simulink model "final_heart_sym2_level5_hdl"  (R2021a)
settings: Solver=FixedStepDiscrete  StartTime=0.0  StopTime=10.0  RelTol=1e-3
undefined symbols (not defined in the file or in its folder): lambda2
(part 2 of 3)

== system final_heart_sym2_level5_hdl/DWT_Sym2_Level5/1st_Level_Decomp4/HiD_Even ==
  In_HiD_e : Inport  OutDataTypeStr=fixdt(0,16,24)  SampleTime=1/44100
  Add : Sum  AccumDataTypeStr=fixdt(1,16,15)  OutDataTypeStr=fixdt(1,16,15)
  Delay : Delay  DelayLength=1  SampleTime=1/44100
  Delay3 : Delay  DelayLength=1  SampleTime=1/44100
  HiD_0 : Constant  Value=-0.482962913  OutDataTypeStr=fixdt(1,16,16)  SampleTime=1/44100
  HiD_2 : Constant  Value=-0.224143868  OutDataTypeStr=fixdt(1,16,17)  SampleTime=1/44100
  Multiply : Product  OutDataTypeStr=fixdt(1,16,15)
  Multiply1 : Product  OutDataTypeStr=fixdt(1,16,15)
  Rate Transition : RateTransition
  Out_HiD_e : Outport  OutDataTypeStr=fixdt(1,16,15)  SampleTime=1/44100  VectorParamsAs1DForOutWhenUnconnected=off
  wires:
  Delay/1 -> Rate Transition/1
  Delay3/1 -> Add/2
  Multiply1/1 -> Delay3/1
  Multiply/1 -> Add/1
  HiD_0/1 -> Multiply/1
  HiD_2/1 -> Multiply1/1
  Add/1 -> Out_HiD_e/1
  In_HiD_e/1 -> Multiply/2, Delay/1
  Rate Transition/1 -> Multiply1/2

== system final_heart_sym2_level5_hdl/DWT_Sym2_Level5/1st_Level_Decomp4/HiD_Odd ==
  In_HiD_o : Inport  OutDataTypeStr=fixdt(0,16,24)  SampleTime=1/44100
  Add : Sum  AccumDataTypeStr=fixdt(1,16,23)  OutDataTypeStr=fixdt(1,16,24)
  Delay : Delay  DelayLength=1  SampleTime=1/44100
  Delay3 : Delay  DelayLength=1  SampleTime=1/44100
  HiD_1 : Constant  Value=0.836516304  OutDataTypeStr=fixdt(0,16,16)  SampleTime=1/44100
  HiD_3 : Constant  Value=-0.129409523  OutDataTypeStr=fixdt(1,16,17)  SampleTime=1/44100
  Multiply : Product  OutDataTypeStr=fixdt(0,16,24)
  Multiply1 : Product  OutDataTypeStr=fixdt(1,16,15)
  Rate Transition : RateTransition
  Out_HiD_o : Outport  OutDataTypeStr=fixdt(1,16,24)  SampleTime=1/44100  VectorParamsAs1DForOutWhenUnconnected=off
  wires:
  Delay/1 -> Rate Transition/1
  Delay3/1 -> Add/2
  Multiply1/1 -> Delay3/1
  Multiply/1 -> Add/1
  HiD_1/1 -> Multiply/1
  HiD_3/1 -> Multiply1/1
  Add/1 -> Out_HiD_o/1
  In_HiD_o/1 -> Delay/1, Multiply/2
  Rate Transition/1 -> Multiply1/2

== system final_heart_sym2_level5_hdl/DWT_Sym2_Level5/1st_Level_Decomp4/LoD_Even ==
  In_LoD_e : Inport  OutDataTypeStr=fixdt(0,16,24)  SampleTime=1/44100
  Add : Sum  AccumDataTypeStr=fixdt(1,16,23)  OutDataTypeStr=fixdt(1,16,24)
  Delay : Delay  DelayLength=1  SampleTime=1/44100
  Delay3 : Delay  DelayLength=1  SampleTime=1/44100
  LoD_0 : Constant  Value=-0.129409523  OutDataTypeStr=fixdt(1,16,17)  SampleTime=1/44100
  LoD_2 : Constant  Value=0.836516304  OutDataTypeStr=fixdt(0,16,16)  SampleTime=1/44100
  Multiply : Product  OutDataTypeStr=fixdt(1,16,15)
  Multiply1 : Product  OutDataTypeStr=fixdt(0,16,24)
  Rate Transition : RateTransition
  Out_LoD_e : Outport  OutDataTypeStr=fixdt(1,16,24)  SampleTime=1/44100  VectorParamsAs1DForOutWhenUnconnected=off
  wires:
  Delay/1 -> Rate Transition/1
  Delay3/1 -> Add/2
  Multiply1/1 -> Delay3/1
  Multiply/1 -> Add/1
  LoD_0/1 -> Multiply/1
  LoD_2/1 -> Multiply1/1
  Add/1 -> Out_LoD_e/1
  In_LoD_e/1 -> Delay/1, Multiply/2
  Rate Transition/1 -> Multiply1/2

== system final_heart_sym2_level5_hdl/DWT_Sym2_Level5/1st_Level_Decomp4/LoD_Odd ==
  In_LoD_o : Inport  OutDataTypeStr=fixdt(0,16,24)  SampleTime=1/44100
  Add : Sum  AccumDataTypeStr=fixdt(0,16,25)  OutDataTypeStr=fixdt(0,16,25)
  Delay : Delay  DelayLength=1  SampleTime=1/44100
  Delay3 : Delay  DelayLength=1  SampleTime=1/44100
  LoD_1 : Constant  Value=0.224143868  OutDataTypeStr=fixdt(0,16,18)  SampleTime=1/44100
  LoD_3 : Constant  Value=0.482962913  OutDataTypeStr=fixdt(0,16,17)  SampleTime=1/44100
  Multiply : Product  OutDataTypeStr=fixdt(0,16,26)
  Multiply1 : Product  OutDataTypeStr=fixdt(0,16,25)
  Rate Transition : RateTransition
  Out_LoD_o : Outport  OutDataTypeStr=fixdt(0,16,25)  SampleTime=1/44100  VectorParamsAs1DForOutWhenUnconnected=off
  wires:
  Delay/1 -> Rate Transition/1
  Delay3/1 -> Add/2
  Multiply1/1 -> Delay3/1
  Multiply/1 -> Add/1
  LoD_1/1 -> Multiply/1
  LoD_3/1 -> Multiply1/1
  Add/1 -> Out_LoD_o/1
  In_LoD_o/1 -> Delay/1, Multiply/2
  Rate Transition/1 -> Multiply1/2

== system final_heart_sym2_level5_hdl/DWT_Sym2_Level5/1st_Level_Recon/HiR_Even ==
  In_HiR_e : Inport  OutDataTypeStr=fixdt(1,16,27)  SampleTime=1/44100
  Add : Sum  AccumDataTypeStr=fixdt(1,16,28)  OutDataTypeStr=fixdt(1,16,28)
  Constant12 : Constant  Value=-0.129409523  OutDataTypeStr=fixdt(1,16,17)  SampleTime=1/44100
  Constant14 : Constant  Value=0.836516304  OutDataTypeStr=fixdt(0,16,16)  SampleTime=1/44100
  Delay : Delay  DelayLength=1  SampleTime=1/44100
  Delay3 : Delay  DelayLength=1  SampleTime=1/44100
  Multiply : Product  OutDataTypeStr=fixdt(1,16,30)
  Multiply1 : Product  OutDataTypeStr=fixdt(1,16,28)
  Rate Transition : RateTransition
  Out_HiR_e : Outport  OutDataTypeStr=fixdt(1,16,28)  SampleTime=1/44100  VectorParamsAs1DForOutWhenUnconnected=off
  wires:
  In_HiR_e/1 -> Multiply/2, Delay/1
  Delay3/1 -> Add/2
  Multiply/1 -> Add/1
  Constant12/1 -> Multiply/1
  Constant14/1 -> Multiply1/1
  Delay/1 -> Rate Transition/1
  Multiply1/1 -> Delay3/1
  Add/1 -> Out_HiR_e/1
  Rate Transition/1 -> Multiply1/2

== system final_heart_sym2_level5_hdl/DWT_Sym2_Level5/1st_Level_Recon/HiR_Odd ==
  In_HiR_o : Inport  OutDataTypeStr=fixdt(1,16,27)  SampleTime=1/44100
  Add : Sum  AccumDataTypeStr=fixdt(1,16,29)  OutDataTypeStr=fixdt(1,16,29)
  Constant13 : Constant  Value=-0.224143868  OutDataTypeStr=fixdt(1,16,17)  SampleTime=1/44100
  Constant15 : Constant  Value=-0.482962913  OutDataTypeStr=fixdt(1,16,16)  SampleTime=1/44100
  Delay : Delay  DelayLength=1  SampleTime=1/44100
  Delay3 : Delay  DelayLength=1  SampleTime=1/44100
  Multiply : Product  OutDataTypeStr=fixdt(1,16,30)
  Multiply1 : Product  OutDataTypeStr=fixdt(1,16,29)
  Rate Transition : RateTransition
  Out_HiR_o : Outport  OutDataTypeStr=fixdt(1,16,29)  SampleTime=1/44100  VectorParamsAs1DForOutWhenUnconnected=off
  wires:
  In_HiR_o/1 -> Multiply/2, Delay/1
  Delay3/1 -> Add/2
  Multiply1/1 -> Delay3/1
  Multiply/1 -> Add/1
  Constant13/1 -> Multiply/1
  Constant15/1 -> Multiply1/1
  Add/1 -> Out_HiR_o/1
  Delay/1 -> Rate Transition/1
  Rate Transition/1 -> Multiply1/2

== system final_heart_sym2_level5_hdl/DWT_Sym2_Level5/1st_Level_Recon/LoR_Even ==
  In_LoR_e : Inport  OutDataTypeStr=fixdt(0,16,24)  SampleTime=1/44100
  Add : Sum  AccumDataTypeStr=fixdt(0,16,25)  OutDataTypeStr=fixdt(0,16,25)
  Constant10 : Constant  Value=0.224143868  OutDataTypeStr=fixdt(0,16,18)  SampleTime=1/44100
  Constant8 : Constant  Value=0.482962913  OutDataTypeStr=fixdt(0,16,17)  SampleTime=1/44100
  Delay : Delay  DelayLength=1  SampleTime=1/44100
  Delay3 : Delay  DelayLength=1  SampleTime=1/44100
  Multiply : Product  OutDataTypeStr=fixdt(0,16,25)
  Multiply1 : Product  OutDataTypeStr=fixdt(0,16,27)
  Rate Transition : RateTransition
  Out_LoR_e : Outport  OutDataTypeStr=fixdt(0,16,25)  SampleTime=1/44100  VectorParamsAs1DForOutWhenUnconnected=off
  wires:
  In_LoR_e/1 -> Multiply/2, Delay/1
  Delay3/1 -> Add/2
  Multiply1/1 -> Delay3/1
  Multiply/1 -> Add/1
  Constant8/1 -> Multiply/1
  Constant10/1 -> Multiply1/1
  Add/1 -> Out_LoR_e/1
  Delay/1 -> Rate Transition/1
  Rate Transition/1 -> Multiply1/2

== system final_heart_sym2_level5_hdl/DWT_Sym2_Level5/1st_Level_Recon/LoR_Odd ==
  In_LoR_o : Inport  OutDataTypeStr=fixdt(0,16,24)  SampleTime=1/44100
  Add : Sum  AccumDataTypeStr=fixdt(1,16,24)  OutDataTypeStr=fixdt(1,16,24)
  Constant11 : Constant  Value=-0.129409523  OutDataTypeStr=fixdt(1,16,17)  SampleTime=1/44100
  Constant9 : Constant  Value=0.836516304  OutDataTypeStr=fixdt(0,16,16)  SampleTime=1/44100
  Delay : Delay  DelayLength=1  SampleTime=1/44100
  Delay3 : Delay  DelayLength=1  SampleTime=1/44100
  Multiply : Product  OutDataTypeStr=fixdt(0,16,25)
  Multiply1 : Product  OutDataTypeStr=fixdt(1,16,15)
  Rate Transition : RateTransition
  Out_HiR_o : Outport  OutDataTypeStr=fixdt(1,16,24)  SampleTime=1/44100  VectorParamsAs1DForOutWhenUnconnected=off
  wires:
  In_LoR_o/1 -> Multiply/2, Delay/1
  Delay3/1 -> Add/2
  Multiply1/1 -> Delay3/1
  Multiply/1 -> Add/1
  Constant9/1 -> Multiply/1
  Constant11/1 -> Multiply1/1
  Add/1 -> Out_HiR_o/1
  Delay/1 -> Rate Transition/1
  Rate Transition/1 -> Multiply1/2

== system final_heart_sym2_level5_hdl/DWT_Sym2_Level5/1st_Level_Recon1/HiR_Even ==
  In_HiR_e : Inport  OutDataTypeStr=fixdt(1,16,27)  SampleTime=1/44100
  Add : Sum  AccumDataTypeStr=fixdt(1,16,28)  OutDataTypeStr=fixdt(1,16,28)
  Constant12 : Constant  Value=-0.129409523  OutDataTypeStr=fixdt(1,16,17)  SampleTime=1/44100
  Constant14 : Constant  Value=0.836516304  OutDataTypeStr=fixdt(0,16,16)  SampleTime=1/44100
  Delay : Delay  DelayLength=1  SampleTime=1/44100
  Delay3 : Delay  DelayLength=1  SampleTime=1/44100
  Multiply : Product  OutDataTypeStr=fixdt(1,16,30)
  Multiply1 : Product  OutDataTypeStr=fixdt(1,16,28)
  Rate Transition : RateTransition
  Out_HiR_e : Outport  OutDataTypeStr=fixdt(1,16,28)  SampleTime=1/44100  VectorParamsAs1DForOutWhenUnconnected=off
  wires:
  In_HiR_e/1 -> Multiply/2, Delay/1
  Delay3/1 -> Add/2
  Multiply/1 -> Add/1
  Constant12/1 -> Multiply/1
  Constant14/1 -> Multiply1/1
  Delay/1 -> Rate Transition/1
  Multiply1/1 -> Delay3/1
  Add/1 -> Out_HiR_e/1
  Rate Transition/1 -> Multiply1/2

== system final_heart_sym2_level5_hdl/DWT_Sym2_Level5/1st_Level_Recon1/HiR_Odd ==
  In_HiR_o : Inport  OutDataTypeStr=fixdt(1,16,27)  SampleTime=1/44100
  Add : Sum  AccumDataTypeStr=fixdt(1,16,29)  OutDataTypeStr=fixdt(1,16,29)
  Constant13 : Constant  Value=-0.224143868  OutDataTypeStr=fixdt(1,16,17)  SampleTime=1/44100
  Constant15 : Constant  Value=-0.482962913  OutDataTypeStr=fixdt(1,16,16)  SampleTime=1/44100
  Delay : Delay  DelayLength=1  SampleTime=1/44100
  Delay3 : Delay  DelayLength=1  SampleTime=1/44100
  Multiply : Product  OutDataTypeStr=fixdt(1,16,30)
  Multiply1 : Product  OutDataTypeStr=fixdt(1,16,29)
  Rate Transition : RateTransition
  Out_HiR_o : Outport  OutDataTypeStr=fixdt(1,16,29)  SampleTime=1/44100  VectorParamsAs1DForOutWhenUnconnected=off
  wires:
  In_HiR_o/1 -> Multiply/2, Delay/1
  Delay3/1 -> Add/2
  Multiply1/1 -> Delay3/1
  Multiply/1 -> Add/1
  Constant13/1 -> Multiply/1
  Constant15/1 -> Multiply1/1
  Add/1 -> Out_HiR_o/1
  Delay/1 -> Rate Transition/1
  Rate Transition/1 -> Multiply1/2

== system final_heart_sym2_level5_hdl/DWT_Sym2_Level5/1st_Level_Recon1/LoR_Even ==
  In_LoR_e : Inport  OutDataTypeStr=fixdt(1,16,23)  SampleTime=1/44100
  Add : Sum  AccumDataTypeStr=fixdt(1,16,24)  OutDataTypeStr=fixdt(1,16,24)
  Constant10 : Constant  Value=0.224143868  OutDataTypeStr=fixdt(0,16,18)  SampleTime=1/44100
  Constant8 : Constant  Value=0.482962913  OutDataTypeStr=fixdt(0,16,17)  SampleTime=1/44100
  Delay : Delay  DelayLength=1  SampleTime=1/44100
  Delay3 : Delay  DelayLength=1  SampleTime=1/44100
  Multiply : Product  OutDataTypeStr=fixdt(1,16,24)
  Multiply1 : Product  OutDataTypeStr=fixdt(1,16,25)
  Rate Transition : RateTransition
  Out_LoR_e : Outport  OutDataTypeStr=fixdt(1,16,24)  SampleTime=1/44100  VectorParamsAs1DForOutWhenUnconnected=off
  wires:
  In_LoR_e/1 -> Multiply/2, Delay/1
  Delay3/1 -> Add/2
  Multiply1/1 -> Delay3/1
  Multiply/1 -> Add/1
  Constant8/1 -> Multiply/1
  Constant10/1 -> Multiply1/1
  Add/1 -> Out_LoR_e/1
  Delay/1 -> Rate Transition/1
  Rate Transition/1 -> Multiply1/2

== system final_heart_sym2_level5_hdl/DWT_Sym2_Level5/1st_Level_Recon1/LoR_Odd ==
  In_LoR_o : Inport  OutDataTypeStr=fixdt(1,16,23)  SampleTime=1/44100
  Add : Sum  AccumDataTypeStr=fixdt(1,16,23)  OutDataTypeStr=fixdt(1,16,24)
  Constant11 : Constant  Value=-0.129409523  OutDataTypeStr=fixdt(1,16,17)  SampleTime=1/44100
  Constant9 : Constant  Value=0.836516304  OutDataTypeStr=fixdt(0,16,16)  SampleTime=1/44100
  Delay : Delay  DelayLength=1  SampleTime=1/44100
  Delay3 : Delay  DelayLength=1  SampleTime=1/44100
  Multiply : Product  OutDataTypeStr=fixdt(1,16,23)
  Multiply1 : Product  OutDataTypeStr=fixdt(1,16,26)
  Rate Transition : RateTransition
  Out_HiR_o : Outport  OutDataTypeStr=fixdt(1,16,24)  SampleTime=1/44100  VectorParamsAs1DForOutWhenUnconnected=off
  wires:
  In_LoR_o/1 -> Multiply/2, Delay/1
  Delay3/1 -> Add/2
  Multiply1/1 -> Delay3/1
  Multiply/1 -> Add/1
  Constant9/1 -> Multiply/1
  Constant11/1 -> Multiply1/1
  Add/1 -> Out_HiR_o/1
  Delay/1 -> Rate Transition/1
  Rate Transition/1 -> Multiply1/2

== system final_heart_sym2_level5_hdl/DWT_Sym2_Level5/1st_Level_Recon2/HiR_Even ==
  In_HiR_e : Inport  OutDataTypeStr=fixdt(1,16,27)  SampleTime=1/44100
  Add : Sum  AccumDataTypeStr=fixdt(1,16,28)  OutDataTypeStr=fixdt(1,16,28)
  Constant12 : Constant  Value=-0.129409523  OutDataTypeStr=fixdt(1,16,17)  SampleTime=1/44100
  Constant14 : Constant  Value=0.836516304  OutDataTypeStr=fixdt(0,16,16)  SampleTime=1/44100
  Delay : Delay  DelayLength=1  SampleTime=1/44100
  Delay3 : Delay  DelayLength=1  SampleTime=1/44100
  Multiply : Product  OutDataTypeStr=fixdt(1,16,30)
  Multiply1 : Product  OutDataTypeStr=fixdt(1,16,28)
  Rate Transition : RateTransition
  Out_HiR_e : Outport  OutDataTypeStr=fixdt(1,16,28)  SampleTime=1/44100  VectorParamsAs1DForOutWhenUnconnected=off
  wires:
  In_HiR_e/1 -> Multiply/2, Delay/1
  Delay3/1 -> Add/2
  Multiply/1 -> Add/1
  Constant12/1 -> Multiply/1
  Constant14/1 -> Multiply1/1
  Delay/1 -> Rate Transition/1
  Multiply1/1 -> Delay3/1
  Add/1 -> Out_HiR_e/1
  Rate Transition/1 -> Multiply1/2

== system final_heart_sym2_level5_hdl/DWT_Sym2_Level5/1st_Level_Recon2/HiR_Odd ==
  In_HiR_o : Inport  OutDataTypeStr=fixdt(1,16,27)  SampleTime=1/44100
  Add : Sum  AccumDataTypeStr=fixdt(1,16,29)  OutDataTypeStr=fixdt(1,16,29)
  Constant13 : Constant  Value=-0.224143868  OutDataTypeStr=fixdt(1,16,17)  SampleTime=1/44100
  Constant15 : Constant  Value=-0.482962913  OutDataTypeStr=fixdt(1,16,16)  SampleTime=1/44100
  Delay : Delay  DelayLength=1  SampleTime=1/44100
  Delay3 : Delay  DelayLength=1  SampleTime=1/44100
  Multiply : Product  OutDataTypeStr=fixdt(1,16,30)
  Multiply1 : Product  OutDataTypeStr=fixdt(1,16,29)
  Rate Transition : RateTransition
  Out_HiR_o : Outport  OutDataTypeStr=fixdt(1,16,29)  SampleTime=1/44100  VectorParamsAs1DForOutWhenUnconnected=off
  wires:
  In_HiR_o/1 -> Multiply/2, Delay/1
  Delay3/1 -> Add/2
  Multiply1/1 -> Delay3/1
  Multiply/1 -> Add/1
  Constant13/1 -> Multiply/1
  Constant15/1 -> Multiply1/1
  Add/1 -> Out_HiR_o/1
  Delay/1 -> Rate Transition/1
  Rate Transition/1 -> Multiply1/2

== system final_heart_sym2_level5_hdl/DWT_Sym2_Level5/1st_Level_Recon2/LoR_Even ==
  In_LoR_e : Inport  OutDataTypeStr=fixdt(1,16,23)  SampleTime=1/44100
  Add : Sum  AccumDataTypeStr=fixdt(1,16,23)  OutDataTypeStr=fixdt(1,16,23)
  Constant10 : Constant  Value=0.224143868  OutDataTypeStr=fixdt(0,16,18)  SampleTime=1/44100
  Constant8 : Constant  Value=0.482962913  OutDataTypeStr=fixdt(0,16,17)  SampleTime=1/44100
  Delay : Delay  DelayLength=1  SampleTime=1/44100
  Delay3 : Delay  DelayLength=1  SampleTime=1/44100
  Multiply : Product  OutDataTypeStr=fixdt(1,16,24)
  Multiply1 : Product  OutDataTypeStr=fixdt(1,16,25)
  Rate Transition : RateTransition
  Out_LoR_e : Outport  OutDataTypeStr=fixdt(1,16,23)  SampleTime=1/44100  VectorParamsAs1DForOutWhenUnconnected=off
  wires:
  In_LoR_e/1 -> Multiply/2, Delay/1
  Delay3/1 -> Add/2
  Multiply1/1 -> Delay3/1
  Multiply/1 -> Add/1
  Constant8/1 -> Multiply/1
  Constant10/1 -> Multiply1/1
  Add/1 -> Out_LoR_e/1
  Delay/1 -> Rate Transition/1
  Rate Transition/1 -> Multiply1/2

== system final_heart_sym2_level5_hdl/DWT_Sym2_Level5/1st_Level_Recon2/LoR_Odd ==
  In_LoR_o : Inport  OutDataTypeStr=fixdt(1,16,23)  SampleTime=1/44100
  Add : Sum  AccumDataTypeStr=fixdt(1,16,23)  OutDataTypeStr=fixdt(1,16,23)
  Constant11 : Constant  Value=-0.129409523  OutDataTypeStr=fixdt(1,16,17)  SampleTime=1/44100
  Constant9 : Constant  Value=0.836516304  OutDataTypeStr=fixdt(0,16,16)  SampleTime=1/44100
  Delay : Delay  DelayLength=1  SampleTime=1/44100
  Delay3 : Delay  DelayLength=1  SampleTime=1/44100
  Multiply : Product  OutDataTypeStr=fixdt(1,16,23)
  Multiply1 : Product  OutDataTypeStr=fixdt(1,16,26)
  Rate Transition : RateTransition
  Out_HiR_o : Outport  OutDataTypeStr=fixdt(1,16,23)  SampleTime=1/44100  VectorParamsAs1DForOutWhenUnconnected=off
  wires:
  In_LoR_o/1 -> Multiply/2, Delay/1
  Delay3/1 -> Add/2
  Multiply1/1 -> Delay3/1
  Multiply/1 -> Add/1
  Constant9/1 -> Multiply/1
  Constant11/1 -> Multiply1/1
  Add/1 -> Out_HiR_o/1
  Delay/1 -> Rate Transition/1
  Rate Transition/1 -> Multiply1/2

== system final_heart_sym2_level5_hdl/DWT_Sym2_Level5/1st_Level_Recon3/HiR_Even ==
  In_HiR_e : Inport  OutDataTypeStr=fixdt(1,16,27)  SampleTime=1/44100
  Add : Sum  AccumDataTypeStr=fixdt(1,16,28)  OutDataTypeStr=fixdt(1,16,28)
  Constant12 : Constant  Value=-0.129409523  OutDataTypeStr=fixdt(1,16,17)  SampleTime=1/44100
  Constant14 : Constant  Value=0.836516304  OutDataTypeStr=fixdt(0,16,16)  SampleTime=1/44100
  Delay : Delay  DelayLength=1  SampleTime=1/44100
  Delay3 : Delay  DelayLength=1  SampleTime=1/44100
  Multiply : Product  OutDataTypeStr=fixdt(1,16,30)
  Multiply1 : Product  OutDataTypeStr=fixdt(1,16,28)
  Rate Transition : RateTransition
  Out_HiR_e : Outport  OutDataTypeStr=fixdt(1,16,28)  SampleTime=1/44100  VectorParamsAs1DForOutWhenUnconnected=off
  wires:
  In_HiR_e/1 -> Multiply/2, Delay/1
  Delay3/1 -> Add/2
  Multiply/1 -> Add/1
  Constant12/1 -> Multiply/1
  Constant14/1 -> Multiply1/1
  Delay/1 -> Rate Transition/1
  Multiply1/1 -> Delay3/1
  Add/1 -> Out_HiR_e/1
  Rate Transition/1 -> Multiply1/2

== system final_heart_sym2_level5_hdl/DWT_Sym2_Level5/1st_Level_Recon3/HiR_Odd ==
  In_HiR_o : Inport  OutDataTypeStr=fixdt(1,16,27)  SampleTime=1/44100
  Add : Sum  AccumDataTypeStr=fixdt(1,16,29)  OutDataTypeStr=fixdt(1,16,29)
  Constant13 : Constant  Value=-0.224143868  OutDataTypeStr=fixdt(1,16,17)  SampleTime=1/44100
  Constant15 : Constant  Value=-0.482962913  OutDataTypeStr=fixdt(1,16,16)  SampleTime=1/44100
  Delay : Delay  DelayLength=1  SampleTime=1/44100
  Delay3 : Delay  DelayLength=1  SampleTime=1/44100
  Multiply : Product  OutDataTypeStr=fixdt(1,16,30)
  Multiply1 : Product  OutDataTypeStr=fixdt(1,16,29)
  Rate Transition : RateTransition
  Out_HiR_o : Outport  OutDataTypeStr=fixdt(1,16,29)  SampleTime=1/44100  VectorParamsAs1DForOutWhenUnconnected=off
  wires:
  In_HiR_o/1 -> Multiply/2, Delay/1
  Delay3/1 -> Add/2
  Multiply1/1 -> Delay3/1
  Multiply/1 -> Add/1
  Constant13/1 -> Multiply/1
  Constant15/1 -> Multiply1/1
  Add/1 -> Out_HiR_o/1
  Delay/1 -> Rate Transition/1
  Rate Transition/1 -> Multiply1/2

== system final_heart_sym2_level5_hdl/DWT_Sym2_Level5/1st_Level_Recon3/LoR_Even ==
  In_LoR_e : Inport  OutDataTypeStr=fixdt(1,16,23)  SampleTime=1/44100
  Add : Sum  AccumDataTypeStr=fixdt(1,16,23)  OutDataTypeStr=fixdt(1,16,23)
  Constant10 : Constant  Value=0.224143868  OutDataTypeStr=fixdt(0,16,18)  SampleTime=1/44100
  Constant8 : Constant  Value=0.482962913  OutDataTypeStr=fixdt(0,16,17)  SampleTime=1/44100
  Delay : Delay  DelayLength=1  SampleTime=1/44100
  Delay3 : Delay  DelayLength=1  SampleTime=1/44100
  Multiply : Product  OutDataTypeStr=fixdt(1,16,24)
  Multiply1 : Product  OutDataTypeStr=fixdt(1,16,25)
  Rate Transition : RateTransition
  Out_LoR_e : Outport  OutDataTypeStr=fixdt(1,16,23)  SampleTime=1/44100  VectorParamsAs1DForOutWhenUnconnected=off
  wires:
  In_LoR_e/1 -> Multiply/2, Delay/1
  Delay3/1 -> Add/2
  Multiply1/1 -> Delay3/1
  Multiply/1 -> Add/1
  Constant8/1 -> Multiply/1
  Constant10/1 -> Multiply1/1
  Add/1 -> Out_LoR_e/1
  Delay/1 -> Rate Transition/1
  Rate Transition/1 -> Multiply1/2

== system final_heart_sym2_level5_hdl/DWT_Sym2_Level5/1st_Level_Recon3/LoR_Odd ==
  In_LoR_o : Inport  OutDataTypeStr=fixdt(1,16,23)  SampleTime=1/44100
  Add : Sum  AccumDataTypeStr=fixdt(1,16,23)  OutDataTypeStr=fixdt(1,16,23)
  Constant11 : Constant  Value=-0.129409523  OutDataTypeStr=fixdt(1,16,17)  SampleTime=1/44100
  Constant9 : Constant  Value=0.836516304  OutDataTypeStr=fixdt(0,16,16)  SampleTime=1/44100
  Delay : Delay  DelayLength=1  SampleTime=1/44100
  Delay3 : Delay  DelayLength=1  SampleTime=1/44100
  Multiply : Product  OutDataTypeStr=fixdt(1,16,23)
  Multiply1 : Product  OutDataTypeStr=fixdt(1,16,26)
  Rate Transition : RateTransition
  Out_HiR_o : Outport  OutDataTypeStr=fixdt(1,16,23)  SampleTime=1/44100  VectorParamsAs1DForOutWhenUnconnected=off
  wires:
  In_LoR_o/1 -> Multiply/2, Delay/1
  Delay3/1 -> Add/2
  Multiply1/1 -> Delay3/1
  Multiply/1 -> Add/1
  Constant9/1 -> Multiply/1
  Constant11/1 -> Multiply1/1
  Add/1 -> Out_HiR_o/1
  Delay/1 -> Rate Transition/1
  Rate Transition/1 -> Multiply1/2

== system final_heart_sym2_level5_hdl/DWT_Sym2_Level5/1st_Level_Recon4/HiR_Even ==
  In_HiR_e : Inport  OutDataTypeStr=fixdt(1,16,28)  SampleTime=1/44100
  Add : Sum  AccumDataTypeStr=fixdt(1,16,28)  OutDataTypeStr=fixdt(1,16,28)
  Constant12 : Constant  Value=-0.129409523  OutDataTypeStr=fixdt(1,16,17)  SampleTime=1/44100
  Constant14 : Constant  Value=0.836516304  OutDataTypeStr=fixdt(0,16,16)  SampleTime=1/44100
  Delay : Delay  DelayLength=1  SampleTime=1/44100
  Delay3 : Delay  DelayLength=1  SampleTime=1/44100
  Multiply : Product  OutDataTypeStr=fixdt(1,16,30)
  Multiply1 : Product  OutDataTypeStr=fixdt(1,16,28)
  Rate Transition : RateTransition
  Out_HiR_e : Outport  OutDataTypeStr=fixdt(1,16,28)  SampleTime=1/44100  VectorParamsAs1DForOutWhenUnconnected=off
  wires:
  In_HiR_e/1 -> Multiply/2, Delay/1
  Delay3/1 -> Add/2
  Multiply/1 -> Add/1
  Constant12/1 -> Multiply/1
  Constant14/1 -> Multiply1/1
  Delay/1 -> Rate Transition/1
  Multiply1/1 -> Delay3/1
  Add/1 -> Out_HiR_e/1
  Rate Transition/1 -> Multiply1/2

== system final_heart_sym2_level5_hdl/DWT_Sym2_Level5/1st_Level_Recon4/HiR_Odd ==
  In_HiR_o : Inport  OutDataTypeStr=fixdt(1,16,28)  SampleTime=1/44100
  Add : Sum  AccumDataTypeStr=fixdt(1,16,28)  OutDataTypeStr=fixdt(1,16,28)
  Constant13 : Constant  Value=-0.224143868  OutDataTypeStr=fixdt(1,16,17)  SampleTime=1/44100
  Constant15 : Constant  Value=-0.482962913  OutDataTypeStr=fixdt(1,16,16)  SampleTime=1/44100
  Delay : Delay  DelayLength=1  SampleTime=1/44100
  Delay3 : Delay  DelayLength=1  SampleTime=1/44100
  Multiply : Product  OutDataTypeStr=fixdt(1,16,30)
  Multiply1 : Product  OutDataTypeStr=fixdt(1,16,29)
  Rate Transition : RateTransition
  Out_HiR_o : Outport  OutDataTypeStr=fixdt(1,16,28)  SampleTime=1/44100  VectorParamsAs1DForOutWhenUnconnected=off
  wires:
  In_HiR_o/1 -> Multiply/2, Delay/1
  Delay3/1 -> Add/2
  Multiply1/1 -> Delay3/1
  Multiply/1 -> Add/1
  Constant13/1 -> Multiply/1
  Constant15/1 -> Multiply1/1
  Add/1 -> Out_HiR_o/1
  Delay/1 -> Rate Transition/1
  Rate Transition/1 -> Multiply1/2

== system final_heart_sym2_level5_hdl/DWT_Sym2_Level5/1st_Level_Recon4/LoR_Even ==
  In_LoR_e : Inport  OutDataTypeStr=fixdt(1,16,22)  SampleTime=1/44100
  Add : Sum  AccumDataTypeStr=fixdt(1,16,23)  OutDataTypeStr=fixdt(1,16,23)
  Constant10 : Constant  Value=0.224143868  OutDataTypeStr=fixdt(0,16,18)  SampleTime=1/44100
  Constant8 : Constant  Value=0.482962913  OutDataTypeStr=fixdt(0,16,17)  SampleTime=1/44100
  Delay : Delay  DelayLength=1  SampleTime=1/44100
  Delay3 : Delay  DelayLength=1  SampleTime=1/44100
  Multiply : Product  OutDataTypeStr=fixdt(1,16,23)
  Multiply1 : Product  OutDataTypeStr=fixdt(1,16,25)
  Rate Transition : RateTransition
  Out_LoR_e : Outport  OutDataTypeStr=fixdt(1,16,23)  SampleTime=1/44100  VectorParamsAs1DForOutWhenUnconnected=off
  wires:
  In_LoR_e/1 -> Multiply/2, Delay/1
  Delay3/1 -> Add/2
  Multiply1/1 -> Delay3/1
  Multiply/1 -> Add/1
  Constant8/1 -> Multiply/1
  Constant10/1 -> Multiply1/1
  Add/1 -> Out_LoR_e/1
  Delay/1 -> Rate Transition/1
  Rate Transition/1 -> Multiply1/2

== system final_heart_sym2_level5_hdl/DWT_Sym2_Level5/1st_Level_Recon4/LoR_Odd ==
  In_LoR_o : Inport  OutDataTypeStr=fixdt(1,16,22)  SampleTime=1/44100
  Add : Sum  AccumDataTypeStr=fixdt(1,16,23)  OutDataTypeStr=fixdt(1,16,23)
  Constant11 : Constant  Value=-0.129409523  OutDataTypeStr=fixdt(1,16,17)  SampleTime=1/44100
  Constant9 : Constant  Value=0.836516304  OutDataTypeStr=fixdt(0,16,16)  SampleTime=1/44100
  Delay : Delay  DelayLength=1  SampleTime=1/44100
  Delay3 : Delay  DelayLength=1  SampleTime=1/44100
  Multiply : Product  OutDataTypeStr=fixdt(1,16,23)
  Multiply1 : Product  OutDataTypeStr=fixdt(1,16,25)
  Rate Transition : RateTransition
  Out_HiR_o : Outport  OutDataTypeStr=fixdt(1,16,23)  SampleTime=1/44100  VectorParamsAs1DForOutWhenUnconnected=off
  wires:
  In_LoR_o/1 -> Multiply/2, Delay/1
  Delay3/1 -> Add/2
  Multiply1/1 -> Delay3/1
  Multiply/1 -> Add/1
  Constant9/1 -> Multiply/1
  Constant11/1 -> Multiply1/1
  Add/1 -> Out_HiR_o/1
  Delay/1 -> Rate Transition/1
  Rate Transition/1 -> Multiply1/2

== system final_heart_sym2_level5_hdl/DWT_Sym2_Level5/Threshold_Estimator/Absolute_Value1 ==
  Signal_w4 : Inport  OutDataTypeStr=fixdt(1,16,26)  SampleTime=1/44100
  Absolute_Switch : Switch  Threshold=1  OutDataTypeStr=fixdt(0,16,27)
  Constant295 : Constant  Value=0  OutDataTypeStr=fixdt(1,16,4)  SampleTime=1/44100
  Gain2 : Gain  Gain=-1  ParamDataTypeStr=fixdt(1,16,15)  OutDataTypeStr=fixdt(0,16,28)
  Relational Operator2 : RelationalOperator  Operator=<  OutDataTypeStr=boolean  RndMeth=Simplest
  Out_Abs : Outport  OutDataTypeStr=fixdt(0,16,27)  SampleTime=1/44100  VectorParamsAs1DForOutWhenUnconnected=off
  wires:
  Absolute_Switch/1 -> Out_Abs/1
  Relational Operator2/1 -> Absolute_Switch/2
  Gain2/1 -> Absolute_Switch/1
  Signal_w4/1 -> Absolute_Switch/3, Relational Operator2/1, Gain2/1
  Constant295/1 -> Relational Operator2/2

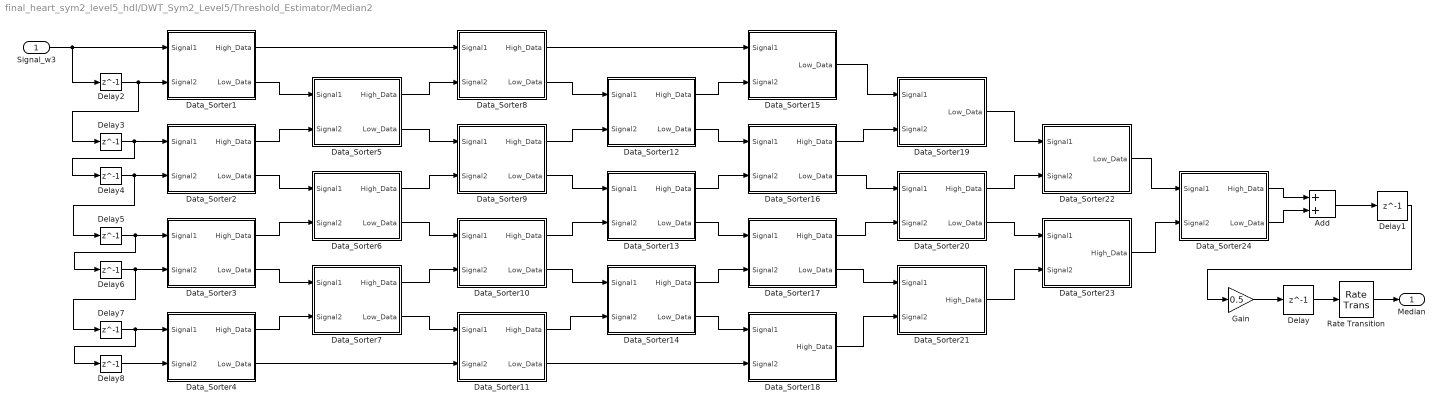
== system final_heart_sym2_level5_hdl/DWT_Sym2_Level5/Threshold_Estimator/Median2 ==
  Signal_w3 : Inport  OutDataTypeStr=fixdt(0,16,27)  SampleTime=1/44100
  Add : Sum  AccumDataTypeStr=fixdt(0,16,26)  OutDataTypeStr=fixdt(0,16,26)
  Data_Sorter1 : Subsystem
  Data_Sorter10 : Subsystem
  Data_Sorter11 : Subsystem
  Data_Sorter12 : Subsystem
  Data_Sorter13 : Subsystem
  Data_Sorter14 : Subsystem
  Data_Sorter15 : Subsystem
  Data_Sorter16 : Subsystem
  Data_Sorter17 : Subsystem
  Data_Sorter18 : Subsystem
  Data_Sorter19 : Subsystem
  Data_Sorter2 : Subsystem
  Data_Sorter20 : Subsystem
  Data_Sorter21 : Subsystem
  Data_Sorter22 : Subsystem
  Data_Sorter23 : Subsystem
  Data_Sorter24 : Subsystem
  Data_Sorter3 : Subsystem
  Data_Sorter4 : Subsystem
  Data_Sorter5 : Subsystem
  Data_Sorter6 : Subsystem
  Data_Sorter7 : Subsystem
  Data_Sorter8 : Subsystem
  Data_Sorter9 : Subsystem
  Delay{,1..8} (9 alike) : Delay  DelayLength=1  SampleTime=1/44100
  Gain : Gain  Gain=0.5  ParamDataTypeStr=fixdt(0,16,16)  OutDataTypeStr=fixdt(0,16,27)
  Rate Transition : RateTransition
  Median : Outport  OutDataTypeStr=fixdt(0,16,27)  SampleTime=1/44100  VectorParamsAs1DForOutWhenUnconnected=off
  wires:
  Data_Sorter4/1(High_Data) -> Data_Sorter7/2(Signal2)
  Delay3/1 -> Data_Sorter2/1(Signal1), Delay4/1
  Signal_w3/1 -> Data_Sorter1/1(Signal1), Delay2/1
  Data_Sorter10/1(High_Data) -> Data_Sorter13/2(Signal2)
  Data_Sorter23/1(High_Data) -> Data_Sorter24/2(Signal2)
  Data_Sorter12/2(Low_Data) -> Data_Sorter16/1(Signal1)
  Delay2/1 -> Delay3/1, Data_Sorter1/2(Signal2)
  Data_Sorter5/1(High_Data) -> Data_Sorter8/2(Signal2)
  Delay/1 -> Rate Transition/1
  Data_Sorter15/1(Low_Data) -> Data_Sorter19/1(Signal1)
  Add/1 -> Delay1/1
  Data_Sorter7/2(Low_Data) -> Data_Sorter11/1(Signal1)
  Data_Sorter24/1(High_Data) -> Add/1
  Data_Sorter1/2(Low_Data) -> Data_Sorter5/1(Signal1)
  Data_Sorter3/1(High_Data) -> Data_Sorter6/2(Signal2)
  Data_Sorter22/1(Low_Data) -> Data_Sorter24/1(Signal1)
  Data_Sorter2/1(High_Data) -> Data_Sorter5/2(Signal2)
  Data_Sorter10/2(Low_Data) -> Data_Sorter14/1(Signal1)
  Delay1/1 -> Gain/1
  Data_Sorter17/2(Low_Data) -> Data_Sorter21/1(Signal1)
  Data_Sorter21/1(High_Data) -> Data_Sorter23/2(Signal2)
  Data_Sorter7/1(High_Data) -> Data_Sorter10/2(Signal2)
  Delay4/1 -> Data_Sorter2/2(Signal2), Delay5/1
  Data_Sorter16/1(High_Data) -> Data_Sorter19/2(Signal2)
  Data_Sorter20/1(High_Data) -> Data_Sorter22/2(Signal2)
  Data_Sorter16/2(Low_Data) -> Data_Sorter20/1(Signal1)
  Data_Sorter3/2(Low_Data) -> Data_Sorter7/1(Signal1)
  Data_Sorter2/2(Low_Data) -> Data_Sorter6/1(Signal1)
  Data_Sorter6/2(Low_Data) -> Data_Sorter10/1(Signal1)
  Data_Sorter19/1(Low_Data) -> Data_Sorter22/1(Signal1)
  Data_Sorter12/1(High_Data) -> Data_Sorter15/2(Signal2)
  Data_Sorter5/2(Low_Data) -> Data_Sorter9/1(Signal1)
  Data_Sorter24/2(Low_Data) -> Add/2
  Data_Sorter17/1(High_Data) -> Data_Sorter20/2(Signal2)
  Data_Sorter13/1(High_Data) -> Data_Sorter16/2(Signal2)
  Data_Sorter11/1(High_Data) -> Data_Sorter14/2(Signal2)
  Delay8/1 -> Data_Sorter4/2(Signal2)
  Data_Sorter8/2(Low_Data) -> Data_Sorter12/1(Signal1)
  Delay6/1 -> Data_Sorter3/2(Signal2), Delay7/1
  Data_Sorter9/2(Low_Data) -> Data_Sorter13/1(Signal1)
  Data_Sorter4/2(Low_Data) -> Data_Sorter11/2(Signal2)
  Data_Sorter9/1(High_Data) -> Data_Sorter12/2(Signal2)
  Data_Sorter14/2(Low_Data) -> Data_Sorter18/1(Signal1)
  Delay5/1 -> Data_Sorter3/1(Signal1), Delay6/1
  Delay7/1 -> Data_Sorter4/1(Signal1), Delay8/1
  Data_Sorter1/1(High_Data) -> Data_Sorter8/1(Signal1)
  Data_Sorter8/1(High_Data) -> Data_Sorter15/1(Signal1)
  Data_Sorter14/1(High_Data) -> Data_Sorter17/2(Signal2)
  Data_Sorter6/1(High_Data) -> Data_Sorter9/2(Signal2)
  Data_Sorter20/2(Low_Data) -> Data_Sorter23/1(Signal1)
  Data_Sorter11/2(Low_Data) -> Data_Sorter18/2(Signal2)
  Data_Sorter13/2(Low_Data) -> Data_Sorter17/1(Signal1)
  Gain/1 -> Delay/1
  Data_Sorter18/1(High_Data) -> Data_Sorter21/2(Signal2)
  Rate Transition/1 -> Median/1

== system final_heart_sym2_level5_hdl/DWT_Sym2_Level5/Threshold_Estimator/Median2/Data_Sorter1 ==
  Signal1 : Inport  OutDataTypeStr=fixdt(0,16,27)  SampleTime=1/44100
  Signal2 : Inport  Port=2  OutDataTypeStr=fixdt(0,16,27)  SampleTime=1/44100
  Data_Sorter_Switch : Switch  OutDataTypeStr=fixdt(0,16,27)
  Data_Sorter_Switch1 : Switch  Threshold=1  OutDataTypeStr=fixdt(0,16,27)
  Delay1 : Delay  DelayLength=1  SampleTime=1/44100
  Delay2 : Delay  DelayLength=1  SampleTime=1/44100
  Relational Operator2 : RelationalOperator  Operator=<  OutDataTypeStr=boolean  RndMeth=Simplest
  High_Data : Outport  OutDataTypeStr=fixdt(0,16,27)  SampleTime=1/44100  VectorParamsAs1DForOutWhenUnconnected=off
  Low_Data : Outport  Port=2  OutDataTypeStr=fixdt(0,16,27)  SampleTime=1/44100  VectorParamsAs1DForOutWhenUnconnected=off
  wires:
  Signal1/1 -> Data_Sorter_Switch/3, Data_Sorter_Switch/1, Relational Operator2/1
  Relational Operator2/1 -> Data_Sorter_Switch1/2, Data_Sorter_Switch/2
  Signal2/1 -> Data_Sorter_Switch1/1, Data_Sorter_Switch1/3, Relational Operator2/2
  Data_Sorter_Switch1/1 -> Delay2/1
  Delay2/1 -> Low_Data/1
  Data_Sorter_Switch/1 -> Delay1/1
  Delay1/1 -> High_Data/1

== system final_heart_sym2_level5_hdl/DWT_Sym2_Level5/Threshold_Estimator/Median2/Data_Sorter10 ==
  Signal1 : Inport  OutDataTypeStr=fixdt(0,16,27)  SampleTime=1/44100
  Signal2 : Inport  Port=2  OutDataTypeStr=fixdt(0,16,27)  SampleTime=1/44100
  Data_Sorter_Switch : Switch  OutDataTypeStr=fixdt(0,16,27)
  Data_Sorter_Switch1 : Switch  Threshold=1  OutDataTypeStr=fixdt(0,16,27)
  Delay1 : Delay  DelayLength=1  SampleTime=1/44100
  Delay2 : Delay  DelayLength=1  SampleTime=1/44100
  Relational Operator2 : RelationalOperator  Operator=<  OutDataTypeStr=boolean  RndMeth=Simplest
  High_Data : Outport  OutDataTypeStr=fixdt(0,16,27)  SampleTime=1/44100  VectorParamsAs1DForOutWhenUnconnected=off
  Low_Data : Outport  Port=2  OutDataTypeStr=fixdt(0,16,27)  SampleTime=1/44100  VectorParamsAs1DForOutWhenUnconnected=off
  wires:
  Signal1/1 -> Data_Sorter_Switch/3, Data_Sorter_Switch/1, Relational Operator2/1
  Relational Operator2/1 -> Data_Sorter_Switch1/2, Data_Sorter_Switch/2
  Signal2/1 -> Data_Sorter_Switch1/1, Data_Sorter_Switch1/3, Relational Operator2/2
  Data_Sorter_Switch1/1 -> Delay2/1
  Delay2/1 -> Low_Data/1
  Data_Sorter_Switch/1 -> Delay1/1
  Delay1/1 -> High_Data/1

== system final_heart_sym2_level5_hdl/DWT_Sym2_Level5/Threshold_Estimator/Median2/Data_Sorter11 ==
  Signal1 : Inport  OutDataTypeStr=fixdt(0,16,27)  SampleTime=1/44100
  Signal2 : Inport  Port=2  OutDataTypeStr=fixdt(0,16,27)  SampleTime=1/44100
  Data_Sorter_Switch : Switch  OutDataTypeStr=fixdt(0,16,27)
  Data_Sorter_Switch1 : Switch  Threshold=1  OutDataTypeStr=fixdt(0,16,27)
  Delay1 : Delay  DelayLength=1  SampleTime=1/44100
  Delay2 : Delay  DelayLength=1  SampleTime=1/44100
  Relational Operator2 : RelationalOperator  Operator=<  OutDataTypeStr=boolean  RndMeth=Simplest
  High_Data : Outport  OutDataTypeStr=fixdt(0,16,27)  SampleTime=1/44100  VectorParamsAs1DForOutWhenUnconnected=off
  Low_Data : Outport  Port=2  OutDataTypeStr=fixdt(0,16,27)  SampleTime=1/44100  VectorParamsAs1DForOutWhenUnconnected=off
  wires:
  Signal1/1 -> Data_Sorter_Switch/3, Data_Sorter_Switch/1, Relational Operator2/1
  Relational Operator2/1 -> Data_Sorter_Switch1/2, Data_Sorter_Switch/2
  Signal2/1 -> Data_Sorter_Switch1/1, Data_Sorter_Switch1/3, Relational Operator2/2
  Data_Sorter_Switch1/1 -> Delay2/1
  Delay2/1 -> Low_Data/1
  Data_Sorter_Switch/1 -> Delay1/1
  Delay1/1 -> High_Data/1

== system final_heart_sym2_level5_hdl/DWT_Sym2_Level5/Threshold_Estimator/Median2/Data_Sorter12 ==
  Signal1 : Inport  OutDataTypeStr=fixdt(0,16,27)  SampleTime=1/44100
  Signal2 : Inport  Port=2  OutDataTypeStr=fixdt(0,16,27)  SampleTime=1/44100
  Data_Sorter_Switch : Switch  OutDataTypeStr=fixdt(0,16,27)
  Data_Sorter_Switch1 : Switch  Threshold=1  OutDataTypeStr=fixdt(0,16,27)
  Delay1 : Delay  DelayLength=1  SampleTime=1/44100
  Delay2 : Delay  DelayLength=1  SampleTime=1/44100
  Relational Operator2 : RelationalOperator  Operator=<  OutDataTypeStr=boolean  RndMeth=Simplest
  High_Data : Outport  OutDataTypeStr=fixdt(0,16,27)  SampleTime=1/44100  VectorParamsAs1DForOutWhenUnconnected=off
  Low_Data : Outport  Port=2  OutDataTypeStr=fixdt(0,16,27)  SampleTime=1/44100  VectorParamsAs1DForOutWhenUnconnected=off
  wires:
  Signal1/1 -> Data_Sorter_Switch/3, Data_Sorter_Switch/1, Relational Operator2/1
  Relational Operator2/1 -> Data_Sorter_Switch1/2, Data_Sorter_Switch/2
  Signal2/1 -> Data_Sorter_Switch1/1, Data_Sorter_Switch1/3, Relational Operator2/2
  Data_Sorter_Switch1/1 -> Delay2/1
  Delay2/1 -> Low_Data/1
  Data_Sorter_Switch/1 -> Delay1/1
  Delay1/1 -> High_Data/1

== system final_heart_sym2_level5_hdl/DWT_Sym2_Level5/Threshold_Estimator/Median2/Data_Sorter13 ==
  Signal1 : Inport  OutDataTypeStr=fixdt(0,16,27)  SampleTime=1/44100
  Signal2 : Inport  Port=2  OutDataTypeStr=fixdt(0,16,27)  SampleTime=1/44100
  Data_Sorter_Switch : Switch  OutDataTypeStr=fixdt(0,16,27)
  Data_Sorter_Switch1 : Switch  Threshold=1  OutDataTypeStr=fixdt(0,16,27)
  Delay1 : Delay  DelayLength=1  SampleTime=1/44100
  Delay2 : Delay  DelayLength=1  SampleTime=1/44100
  Relational Operator2 : RelationalOperator  Operator=<  OutDataTypeStr=boolean  RndMeth=Simplest
  High_Data : Outport  OutDataTypeStr=fixdt(0,16,27)  SampleTime=1/44100  VectorParamsAs1DForOutWhenUnconnected=off
  Low_Data : Outport  Port=2  OutDataTypeStr=fixdt(0,16,27)  SampleTime=1/44100  VectorParamsAs1DForOutWhenUnconnected=off
  wires:
  Signal1/1 -> Data_Sorter_Switch/3, Data_Sorter_Switch/1, Relational Operator2/1
  Relational Operator2/1 -> Data_Sorter_Switch1/2, Data_Sorter_Switch/2
  Signal2/1 -> Data_Sorter_Switch1/1, Data_Sorter_Switch1/3, Relational Operator2/2
  Data_Sorter_Switch1/1 -> Delay2/1
  Delay2/1 -> Low_Data/1
  Data_Sorter_Switch/1 -> Delay1/1
  Delay1/1 -> High_Data/1

== system final_heart_sym2_level5_hdl/DWT_Sym2_Level5/Threshold_Estimator/Median2/Data_Sorter14 ==
  Signal1 : Inport  OutDataTypeStr=fixdt(0,16,27)  SampleTime=1/44100
  Signal2 : Inport  Port=2  OutDataTypeStr=fixdt(0,16,27)  SampleTime=1/44100
  Data_Sorter_Switch : Switch  OutDataTypeStr=fixdt(0,16,27)
  Data_Sorter_Switch1 : Switch  Threshold=1  OutDataTypeStr=fixdt(0,16,27)
  Delay1 : Delay  DelayLength=1  SampleTime=1/44100
  Delay2 : Delay  DelayLength=1  SampleTime=1/44100
  Relational Operator2 : RelationalOperator  Operator=<  OutDataTypeStr=boolean  RndMeth=Simplest
  High_Data : Outport  OutDataTypeStr=fixdt(0,16,27)  SampleTime=1/44100  VectorParamsAs1DForOutWhenUnconnected=off
  Low_Data : Outport  Port=2  OutDataTypeStr=fixdt(0,16,27)  SampleTime=1/44100  VectorParamsAs1DForOutWhenUnconnected=off
  wires:
  Signal1/1 -> Data_Sorter_Switch/3, Data_Sorter_Switch/1, Relational Operator2/1
  Relational Operator2/1 -> Data_Sorter_Switch1/2, Data_Sorter_Switch/2
  Signal2/1 -> Data_Sorter_Switch1/1, Data_Sorter_Switch1/3, Relational Operator2/2
  Data_Sorter_Switch1/1 -> Delay2/1
  Delay2/1 -> Low_Data/1
  Data_Sorter_Switch/1 -> Delay1/1
  Delay1/1 -> High_Data/1

== system final_heart_sym2_level5_hdl/DWT_Sym2_Level5/Threshold_Estimator/Median2/Data_Sorter15 ==
  Signal1 : Inport  OutDataTypeStr=fixdt(0,16,27)  SampleTime=1/44100
  Signal2 : Inport  Port=2  OutDataTypeStr=fixdt(0,16,27)  SampleTime=1/44100
  Data_Sorter_Switch1 : Switch  Threshold=1  OutDataTypeStr=fixdt(0,16,27)
  Delay2 : Delay  DelayLength=1  SampleTime=1/44100
  Relational Operator2 : RelationalOperator  Operator=<  OutDataTypeStr=boolean  RndMeth=Simplest
  Low_Data : Outport  OutDataTypeStr=fixdt(0,16,27)  SampleTime=1/44100  VectorParamsAs1DForOutWhenUnconnected=off
  wires:
  Signal1/1 -> Relational Operator2/1
  Relational Operator2/1 -> Data_Sorter_Switch1/2
  Signal2/1 -> Data_Sorter_Switch1/1, Data_Sorter_Switch1/3, Relational Operator2/2
  Data_Sorter_Switch1/1 -> Delay2/1
  Delay2/1 -> Low_Data/1

== system final_heart_sym2_level5_hdl/DWT_Sym2_Level5/Threshold_Estimator/Median2/Data_Sorter16 ==
  Signal1 : Inport  OutDataTypeStr=fixdt(0,16,27)  SampleTime=1/44100
  Signal2 : Inport  Port=2  OutDataTypeStr=fixdt(0,16,27)  SampleTime=1/44100
  Data_Sorter_Switch : Switch  OutDataTypeStr=fixdt(0,16,27)
  Data_Sorter_Switch1 : Switch  Threshold=1  OutDataTypeStr=fixdt(0,16,27)
  Delay1 : Delay  DelayLength=1  SampleTime=1/44100
  Delay2 : Delay  DelayLength=1  SampleTime=1/44100
  Relational Operator2 : RelationalOperator  Operator=<  OutDataTypeStr=boolean  RndMeth=Simplest
  High_Data : Outport  OutDataTypeStr=fixdt(0,16,27)  SampleTime=1/44100  VectorParamsAs1DForOutWhenUnconnected=off
  Low_Data : Outport  Port=2  OutDataTypeStr=fixdt(0,16,27)  SampleTime=1/44100  VectorParamsAs1DForOutWhenUnconnected=off
  wires:
  Signal1/1 -> Data_Sorter_Switch/3, Data_Sorter_Switch/1, Relational Operator2/1
  Relational Operator2/1 -> Data_Sorter_Switch1/2, Data_Sorter_Switch/2
  Signal2/1 -> Data_Sorter_Switch1/1, Data_Sorter_Switch1/3, Relational Operator2/2
  Data_Sorter_Switch1/1 -> Delay2/1
  Delay2/1 -> Low_Data/1
  Data_Sorter_Switch/1 -> Delay1/1
  Delay1/1 -> High_Data/1

== system final_heart_sym2_level5_hdl/DWT_Sym2_Level5/Threshold_Estimator/Median2/Data_Sorter17 ==
  Signal1 : Inport  OutDataTypeStr=fixdt(0,16,27)  SampleTime=1/44100
  Signal2 : Inport  Port=2  OutDataTypeStr=fixdt(0,16,27)  SampleTime=1/44100
  Data_Sorter_Switch : Switch  OutDataTypeStr=fixdt(0,16,27)
  Data_Sorter_Switch1 : Switch  Threshold=1  OutDataTypeStr=fixdt(0,16,27)
  Delay1 : Delay  DelayLength=1  SampleTime=1/44100
  Delay2 : Delay  DelayLength=1  SampleTime=1/44100
  Relational Operator2 : RelationalOperator  Operator=<  OutDataTypeStr=boolean  RndMeth=Simplest
  High_Data : Outport  OutDataTypeStr=fixdt(0,16,27)  SampleTime=1/44100  VectorParamsAs1DForOutWhenUnconnected=off
  Low_Data : Outport  Port=2  OutDataTypeStr=fixdt(0,16,27)  SampleTime=1/44100  VectorParamsAs1DForOutWhenUnconnected=off
  wires:
  Signal1/1 -> Data_Sorter_Switch/3, Data_Sorter_Switch/1, Relational Operator2/1
  Relational Operator2/1 -> Data_Sorter_Switch1/2, Data_Sorter_Switch/2
  Signal2/1 -> Data_Sorter_Switch1/1, Data_Sorter_Switch1/3, Relational Operator2/2
  Data_Sorter_Switch1/1 -> Delay2/1
  Delay2/1 -> Low_Data/1
  Data_Sorter_Switch/1 -> Delay1/1
  Delay1/1 -> High_Data/1

== system final_heart_sym2_level5_hdl/DWT_Sym2_Level5/Threshold_Estimator/Median2/Data_Sorter18 ==
  Signal1 : Inport  OutDataTypeStr=fixdt(0,16,27)  SampleTime=1/44100
  Signal2 : Inport  Port=2  OutDataTypeStr=fixdt(0,16,27)  SampleTime=1/44100
  Data_Sorter_Switch : Switch  OutDataTypeStr=fixdt(0,16,27)
  Delay1 : Delay  DelayLength=1  SampleTime=1/44100
  Relational Operator2 : RelationalOperator  Operator=<  OutDataTypeStr=boolean  RndMeth=Simplest
  High_Data : Outport  OutDataTypeStr=fixdt(0,16,27)  SampleTime=1/44100  VectorParamsAs1DForOutWhenUnconnected=off
  wires:
  Signal1/1 -> Data_Sorter_Switch/3, Data_Sorter_Switch/1, Relational Operator2/1
  Relational Operator2/1 -> Data_Sorter_Switch/2
  Signal2/1 -> Relational Operator2/2
  Data_Sorter_Switch/1 -> Delay1/1
  Delay1/1 -> High_Data/1

== system final_heart_sym2_level5_hdl/DWT_Sym2_Level5/Threshold_Estimator/Median2/Data_Sorter19 ==
  Signal1 : Inport  OutDataTypeStr=fixdt(0,16,27)  SampleTime=1/44100
  Signal2 : Inport  Port=2  OutDataTypeStr=fixdt(0,16,27)  SampleTime=1/44100
  Data_Sorter_Switch1 : Switch  Threshold=1  OutDataTypeStr=fixdt(0,16,27)
  Delay2 : Delay  DelayLength=1  SampleTime=1/44100
  Relational Operator2 : RelationalOperator  Operator=<  OutDataTypeStr=boolean  RndMeth=Simplest
  Low_Data : Outport  OutDataTypeStr=fixdt(0,16,27)  SampleTime=1/44100  VectorParamsAs1DForOutWhenUnconnected=off
  wires:
  Signal1/1 -> Relational Operator2/1
  Relational Operator2/1 -> Data_Sorter_Switch1/2
  Signal2/1 -> Data_Sorter_Switch1/1, Data_Sorter_Switch1/3, Relational Operator2/2
  Data_Sorter_Switch1/1 -> Delay2/1
  Delay2/1 -> Low_Data/1

== system final_heart_sym2_level5_hdl/DWT_Sym2_Level5/Threshold_Estimator/Median2/Data_Sorter2 ==
  Signal1 : Inport  OutDataTypeStr=fixdt(0,16,27)  SampleTime=1/44100
  Signal2 : Inport  Port=2  OutDataTypeStr=fixdt(0,16,27)  SampleTime=1/44100
  Data_Sorter_Switch : Switch  OutDataTypeStr=fixdt(0,16,27)
  Data_Sorter_Switch1 : Switch  Threshold=1  OutDataTypeStr=fixdt(0,16,27)
  Delay1 : Delay  DelayLength=1  SampleTime=1/44100
  Delay2 : Delay  DelayLength=1  SampleTime=1/44100
  Relational Operator2 : RelationalOperator  Operator=<  OutDataTypeStr=boolean  RndMeth=Simplest
  High_Data : Outport  OutDataTypeStr=fixdt(0,16,27)  SampleTime=1/44100  VectorParamsAs1DForOutWhenUnconnected=off
  Low_Data : Outport  Port=2  OutDataTypeStr=fixdt(0,16,27)  SampleTime=1/44100  VectorParamsAs1DForOutWhenUnconnected=off
  wires:
  Signal1/1 -> Data_Sorter_Switch/3, Data_Sorter_Switch/1, Relational Operator2/1
  Relational Operator2/1 -> Data_Sorter_Switch1/2, Data_Sorter_Switch/2
  Signal2/1 -> Data_Sorter_Switch1/1, Data_Sorter_Switch1/3, Relational Operator2/2
  Data_Sorter_Switch1/1 -> Delay2/1
  Delay2/1 -> Low_Data/1
  Data_Sorter_Switch/1 -> Delay1/1
  Delay1/1 -> High_Data/1

== system final_heart_sym2_level5_hdl/DWT_Sym2_Level5/Threshold_Estimator/Median2/Data_Sorter20 ==
  Signal1 : Inport  OutDataTypeStr=fixdt(0,16,27)  SampleTime=1/44100
  Signal2 : Inport  Port=2  OutDataTypeStr=fixdt(0,16,27)  SampleTime=1/44100
  Data_Sorter_Switch : Switch  OutDataTypeStr=fixdt(0,16,27)
  Data_Sorter_Switch1 : Switch  Threshold=1  OutDataTypeStr=fixdt(0,16,27)
  Delay1 : Delay  DelayLength=1  SampleTime=1/44100
  Delay2 : Delay  DelayLength=1  SampleTime=1/44100
  Relational Operator2 : RelationalOperator  Operator=<  OutDataTypeStr=boolean  RndMeth=Simplest
  High_Data : Outport  OutDataTypeStr=fixdt(0,16,27)  SampleTime=1/44100  VectorParamsAs1DForOutWhenUnconnected=off
  Low_Data : Outport  Port=2  OutDataTypeStr=fixdt(0,16,27)  SampleTime=1/44100  VectorParamsAs1DForOutWhenUnconnected=off
  wires:
  Signal1/1 -> Data_Sorter_Switch/3, Data_Sorter_Switch/1, Relational Operator2/1
  Relational Operator2/1 -> Data_Sorter_Switch1/2, Data_Sorter_Switch/2
  Signal2/1 -> Data_Sorter_Switch1/1, Data_Sorter_Switch1/3, Relational Operator2/2
  Data_Sorter_Switch1/1 -> Delay2/1
  Delay2/1 -> Low_Data/1
  Data_Sorter_Switch/1 -> Delay1/1
  Delay1/1 -> High_Data/1

== system final_heart_sym2_level5_hdl/DWT_Sym2_Level5/Threshold_Estimator/Median2/Data_Sorter21 ==
  Signal1 : Inport  OutDataTypeStr=fixdt(0,16,27)  SampleTime=1/44100
  Signal2 : Inport  Port=2  OutDataTypeStr=fixdt(0,16,27)  SampleTime=1/44100
  Data_Sorter_Switch : Switch  OutDataTypeStr=fixdt(0,16,27)
  Delay1 : Delay  DelayLength=1  SampleTime=1/44100
  Relational Operator2 : RelationalOperator  Operator=<  OutDataTypeStr=boolean  RndMeth=Simplest
  High_Data : Outport  OutDataTypeStr=fixdt(0,16,27)  SampleTime=1/44100  VectorParamsAs1DForOutWhenUnconnected=off
  wires:
  Signal1/1 -> Data_Sorter_Switch/3, Data_Sorter_Switch/1, Relational Operator2/1
  Relational Operator2/1 -> Data_Sorter_Switch/2
  Signal2/1 -> Relational Operator2/2
  Data_Sorter_Switch/1 -> Delay1/1
  Delay1/1 -> High_Data/1

== system final_heart_sym2_level5_hdl/DWT_Sym2_Level5/Threshold_Estimator/Median2/Data_Sorter22 ==
  Signal1 : Inport  OutDataTypeStr=fixdt(0,16,27)  SampleTime=1/44100
  Signal2 : Inport  Port=2  OutDataTypeStr=fixdt(0,16,27)  SampleTime=1/44100
  Data_Sorter_Switch1 : Switch  Threshold=1  OutDataTypeStr=fixdt(0,16,27)
  Delay2 : Delay  DelayLength=1  SampleTime=1/44100
  Relational Operator2 : RelationalOperator  Operator=<  OutDataTypeStr=boolean  RndMeth=Simplest
  Low_Data : Outport  OutDataTypeStr=fixdt(0,16,27)  SampleTime=1/44100  VectorParamsAs1DForOutWhenUnconnected=off
  wires:
  Signal1/1 -> Relational Operator2/1
  Relational Operator2/1 -> Data_Sorter_Switch1/2
  Signal2/1 -> Data_Sorter_Switch1/1, Data_Sorter_Switch1/3, Relational Operator2/2
  Data_Sorter_Switch1/1 -> Delay2/1
  Delay2/1 -> Low_Data/1

== system final_heart_sym2_level5_hdl/DWT_Sym2_Level5/Threshold_Estimator/Median2/Data_Sorter23 ==
  Signal1 : Inport  OutDataTypeStr=fixdt(0,16,27)  SampleTime=1/44100
  Signal2 : Inport  Port=2  OutDataTypeStr=fixdt(0,16,27)  SampleTime=1/44100
  Data_Sorter_Switch : Switch  OutDataTypeStr=fixdt(0,16,27)
  Delay1 : Delay  DelayLength=1  SampleTime=1/44100
  Relational Operator2 : RelationalOperator  Operator=<  OutDataTypeStr=boolean  RndMeth=Simplest
  High_Data : Outport  OutDataTypeStr=fixdt(0,16,27)  SampleTime=1/44100  VectorParamsAs1DForOutWhenUnconnected=off
  wires:
  Signal1/1 -> Data_Sorter_Switch/3, Data_Sorter_Switch/1, Relational Operator2/1
  Relational Operator2/1 -> Data_Sorter_Switch/2
  Signal2/1 -> Relational Operator2/2
  Data_Sorter_Switch/1 -> Delay1/1
  Delay1/1 -> High_Data/1

== system final_heart_sym2_level5_hdl/DWT_Sym2_Level5/Threshold_Estimator/Median2/Data_Sorter24 ==
  Signal1 : Inport  OutDataTypeStr=fixdt(0,16,27)  SampleTime=1/44100
  Signal2 : Inport  Port=2  OutDataTypeStr=fixdt(0,16,27)  SampleTime=1/44100
  Data_Sorter_Switch : Switch  OutDataTypeStr=fixdt(0,16,27)
  Data_Sorter_Switch1 : Switch  Threshold=1  OutDataTypeStr=fixdt(0,16,27)
  Delay1 : Delay  DelayLength=1  SampleTime=1/44100
  Delay2 : Delay  DelayLength=1  SampleTime=1/44100
  Relational Operator2 : RelationalOperator  Operator=<  OutDataTypeStr=boolean  RndMeth=Simplest
  High_Data : Outport  OutDataTypeStr=fixdt(0,16,27)  SampleTime=1/44100  VectorParamsAs1DForOutWhenUnconnected=off
  Low_Data : Outport  Port=2  OutDataTypeStr=fixdt(0,16,27)  SampleTime=1/44100  VectorParamsAs1DForOutWhenUnconnected=off
  wires:
  Signal1/1 -> Data_Sorter_Switch/3, Data_Sorter_Switch/1, Relational Operator2/1
  Relational Operator2/1 -> Data_Sorter_Switch1/2, Data_Sorter_Switch/2
  Signal2/1 -> Data_Sorter_Switch1/1, Data_Sorter_Switch1/3, Relational Operator2/2
  Data_Sorter_Switch1/1 -> Delay2/1
  Delay2/1 -> Low_Data/1
  Data_Sorter_Switch/1 -> Delay1/1
  Delay1/1 -> High_Data/1

== system final_heart_sym2_level5_hdl/DWT_Sym2_Level5/Threshold_Estimator/Median2/Data_Sorter3 ==
  Signal1 : Inport  OutDataTypeStr=fixdt(0,16,27)  SampleTime=1/44100
  Signal2 : Inport  Port=2  OutDataTypeStr=fixdt(0,16,27)  SampleTime=1/44100
  Data_Sorter_Switch : Switch  OutDataTypeStr=fixdt(0,16,27)
  Data_Sorter_Switch1 : Switch  Threshold=1  OutDataTypeStr=fixdt(0,16,27)
  Delay1 : Delay  DelayLength=1  SampleTime=1/44100
  Delay2 : Delay  DelayLength=1  SampleTime=1/44100
  Relational Operator2 : RelationalOperator  Operator=<  OutDataTypeStr=boolean  RndMeth=Simplest
  High_Data : Outport  OutDataTypeStr=fixdt(0,16,27)  SampleTime=1/44100  VectorParamsAs1DForOutWhenUnconnected=off
  Low_Data : Outport  Port=2  OutDataTypeStr=fixdt(0,16,27)  SampleTime=1/44100  VectorParamsAs1DForOutWhenUnconnected=off
  wires:
  Signal1/1 -> Data_Sorter_Switch/3, Data_Sorter_Switch/1, Relational Operator2/1
  Relational Operator2/1 -> Data_Sorter_Switch1/2, Data_Sorter_Switch/2
  Signal2/1 -> Data_Sorter_Switch1/1, Data_Sorter_Switch1/3, Relational Operator2/2
  Data_Sorter_Switch1/1 -> Delay2/1
  Delay2/1 -> Low_Data/1
  Data_Sorter_Switch/1 -> Delay1/1
  Delay1/1 -> High_Data/1
